simulink library "tp333079"  (Simulink 5.0)
values from neighbouring files (symbols this model uses):
  b = 1    [main_flock3.m]    (also in main_flock4.m; params_flocking_ros.m)
undefined symbols (not defined in the file or in its folder): AC, AlphaBnd, BetaBnd, CDda, CDde, CDdf, CDdr, CDM, CDmin, CGempty, CGgross, CL0, CLa, CLalphadot, Clbeta, Clda, CLde, CLdf, Cldr, CLM, CLmind, Clp, CLq, Clr, Cm0, Cma, Cmalphadot, Cmde, Cmdf, CmM, Cmq, Cnbeta, Cnda, Cndr, Cnp, Cnr, CP, CT, CYbeta, CYda, CYdr, CYp, CYr, Displacement, dmy, Engine, EulerIni, FuelFlow, FuelIni, J, Jempty, Jeng, Jgross, Jprop, MAC, MAP, MAPLim, MassIni, MaxPower, mempty ... (+26)
libraries: aerosimlib x325, simulink3 x42
(part 5 of 11)

== system tp333079/Transformations/Body-Inertial DCM From Euler Angles ==
  note: Sources
  note: Assemble Body-Inertial DCM
  note: Output
  note: Attitude trigonometry
  Euler : Inport  Port=1  PortDimensions=[3 1]  SampleTime=-1  DataType=auto
      settings: SignalType=auto
  -sin(theta) : Gain  Gain=-1  Multiplication=Element-wise(K.*u)  SaturateOnIntegerOverflow=on
  Demux : Demux  Outputs=3  BusSelectionMode=off
  Math Function : Math  Operator=transpose  OutputSignalType=auto
  Rbi Matrix : simulink3/Signals & Systems/Matrix Concatenation  numInports=3  catMethod=Horizontal
  Rbi Col1 : simulink3/Signals & Systems/Matrix Concatenation  numInports=3  catMethod=Vertical
  Rbi Col2 : simulink3/Signals & Systems/Matrix Concatenation  numInports=3  catMethod=Vertical
  Rbi Col3 : simulink3/Signals & Systems/Matrix Concatenation  numInports=3  catMethod=Vertical
  Sum2 : Sum  Inputs=+-  SaturateOnIntegerOverflow=on
  Sum3 : Sum  Inputs=++  SaturateOnIntegerOverflow=on
  Sum4 : Sum  Inputs=++  SaturateOnIntegerOverflow=on
  Sum5 : Sum  Inputs=+-  SaturateOnIntegerOverflow=on
  cos(phi) : Trigonometry  Operator=cos  OutputSignalType=auto
  cos(phi)cos(psi) : Product  Inputs=2  Multiplication=Element-wise(.*)  SaturateOnIntegerOverflow=on
  cos(phi)cos(theta) : Product  Inputs=2  Multiplication=Element-wise(.*)  SaturateOnIntegerOverflow=on
  cos(phi)sin(psi) : Product  Inputs=2  Multiplication=Element-wise(.*)  SaturateOnIntegerOverflow=on
  cos(phi)sin(theta)cos(psi) : Product  Inputs=3  Multiplication=Element-wise(.*)  SaturateOnIntegerOverflow=on
  cos(phi)sin(theta)sin(psi) : Product  Inputs=3  Multiplication=Element-wise(.*)  SaturateOnIntegerOverflow=on
  cos(psi) : Trigonometry  Operator=cos  OutputSignalType=auto
  cos(theta) : Trigonometry  Operator=cos  OutputSignalType=auto
  cos(theta)cos(psi) : Product  Inputs=2  Multiplication=Element-wise(.*)  SaturateOnIntegerOverflow=on
  cos(theta)sin(psi) : Product  Inputs=2  Multiplication=Element-wise(.*)  SaturateOnIntegerOverflow=on
  sin(phi) : Trigonometry  Operator=sin  OutputSignalType=auto
  sin(phi)cos(psi) : Product  Inputs=2  Multiplication=Element-wise(.*)  SaturateOnIntegerOverflow=on
  sin(phi)cos(theta) : Product  Inputs=2  Multiplication=Element-wise(.*)  SaturateOnIntegerOverflow=on
  sin(phi)sin(psi) : Product  Inputs=2  Multiplication=Element-wise(.*)  SaturateOnIntegerOverflow=on
  sin(phi)sin(theta)cos(psi) : Product  Inputs=3  Multiplication=Element-wise(.*)  SaturateOnIntegerOverflow=on
  sin(psi) : Trigonometry  Operator=sin  OutputSignalType=auto
  sin(theta) : Trigonometry  Operator=sin  OutputSignalType=auto
  DCM : Outport  Port=1
  wires:
  Euler/1 -> Demux/1
  Rbi Col1/1 -> Rbi Matrix/1
  Rbi Col2/1 -> Rbi Matrix/2
  Rbi Col3/1 -> Rbi Matrix/3
  Rbi Matrix/1 -> Math Function/1
  Demux/1 -> sin(phi)/1, cos(phi)/1
  Demux/2 -> cos(theta)/1, sin(theta)/1
  Demux/3 -> cos(psi)/1, sin(psi)/1
  sin(phi)/1 -> sin(phi)cos(psi)/1, sin(phi)sin(psi)/1, sin(phi)cos(theta)/1, sin(phi)sin(theta)cos(psi)/1
  cos(phi)/1 -> cos(phi)cos(theta)/1, cos(phi)sin(theta)sin(psi)/1, cos(phi)sin(theta)cos(psi)/1, cos(phi)cos(psi)/1, cos(phi)sin(psi)/1
  sin(theta)/1 -> cos(phi)sin(theta)cos(psi)/2, cos(phi)sin(theta)sin(psi)/2, sin(phi)sin(theta)cos(psi)/2, -sin(theta)/1
  cos(theta)/1 -> cos(phi)cos(theta)/2, sin(phi)cos(theta)/2, cos(theta)sin(psi)/1, cos(theta)cos(psi)/1
  sin(psi)/1 -> cos(phi)sin(theta)sin(psi)/3, sin(phi)sin(psi)/2, cos(phi)sin(psi)/2, cos(theta)sin(psi)/2
  cos(psi)/1 -> sin(phi)cos(psi)/2, cos(phi)sin(theta)cos(psi)/3, cos(phi)cos(psi)/2, sin(phi)sin(theta)cos(psi)/3, cos(theta)cos(psi)/2
  cos(phi)sin(psi)/1 -> Sum2/2
  cos(phi)cos(psi)/1 -> Sum3/2
  sin(phi)sin(theta)cos(psi)/1 -> Sum3/1, Sum2/1
  cos(phi)sin(theta)cos(psi)/1 -> Sum4/1
  sin(phi)sin(psi)/1 -> Sum4/2
  cos(phi)sin(theta)sin(psi)/1 -> Sum5/1
  sin(phi)cos(psi)/1 -> Sum5/2
  cos(theta)cos(psi)/1 -> Rbi Col1/1
  cos(theta)sin(psi)/1 -> Rbi Col1/2
  -sin(theta)/1 -> Rbi Col1/3
  Sum2/1 -> Rbi Col2/1
  Sum3/1 -> Rbi Col2/2
  sin(phi)cos(theta)/1 -> Rbi Col2/3
  Sum4/1 -> Rbi Col3/1
  Sum5/1 -> Rbi Col3/2
  cos(phi)cos(theta)/1 -> Rbi Col3/3
  Math Function/1 -> DCM/1

== system tp333079/Transformations/Body-Inertial DCM From Quaternions ==
  note: Output
  note: Quaternion products
  note: Assemble Body-Inertial DCM
  note: Sources
  Quaternions : Inport  Port=1  PortDimensions=[4 1]  SampleTime=-1  DataType=auto
      settings: SignalType=auto
  Demux : Demux  Outputs=4  BusSelectionMode=off
  Demux1 : Demux  Outputs=4  BusSelectionMode=off
  Gain{,1..5} (6 alike) : Gain  Gain=2  Multiplication=Element-wise(K.*u)  SaturateOnIntegerOverflow=on
  Get DCM : Math  Operator=transpose  OutputSignalType=auto
  Math Function : Math  Operator=square  OutputSignalType=auto
  Rbi Matrix : simulink3/Signals & Systems/Matrix Concatenation  numInports=3  catMethod=Horizontal
  Rbi Col1 : simulink3/Signals & Systems/Matrix Concatenation  numInports=3  catMethod=Vertical
  Rbi Col2 : simulink3/Signals & Systems/Matrix Concatenation  numInports=3  catMethod=Vertical
  Rbi Col3 : simulink3/Signals & Systems/Matrix Concatenation  numInports=3  catMethod=Vertical
  Sum : Sum  Inputs=++--  SaturateOnIntegerOverflow=on
  Sum1 : Sum  Inputs=++  SaturateOnIntegerOverflow=on
  Sum2 : Sum  Inputs=+-  SaturateOnIntegerOverflow=on
  Sum3 : Sum  Inputs=+-  SaturateOnIntegerOverflow=on
  Sum4 : Sum  Inputs=+-+-  SaturateOnIntegerOverflow=on
  Sum5 : Sum  Inputs=++  SaturateOnIntegerOverflow=on
  Sum6 : Sum  Inputs=++  SaturateOnIntegerOverflow=on
  Sum7 : Sum  Inputs=+-  SaturateOnIntegerOverflow=on
  Sum8 : Sum  Inputs=+--+  SaturateOnIntegerOverflow=on
  exe0 : Product  Inputs=2  Multiplication=Element-wise(.*)  SaturateOnIntegerOverflow=on
  exey : Product  Inputs=2  Multiplication=Element-wise(.*)  SaturateOnIntegerOverflow=on
  exez : Product  Inputs=2  Multiplication=Element-wise(.*)  SaturateOnIntegerOverflow=on
  eye0 : Product  Inputs=2  Multiplication=Element-wise(.*)  SaturateOnIntegerOverflow=on
  eyez : Product  Inputs=2  Multiplication=Element-wise(.*)  SaturateOnIntegerOverflow=on
  eze0 : Product  Inputs=2  Multiplication=Element-wise(.*)  SaturateOnIntegerOverflow=on
  DCM : Outport  Port=1
  wires:
  Get DCM/1 -> DCM/1
  Rbi Matrix/1 -> Get DCM/1
  Sum8/1 -> Rbi Col3/3
  Gain5/1 -> Rbi Col3/2
  Gain4/1 -> Rbi Col3/1
  Rbi Col3/1 -> Rbi Matrix/3
  Sum7/1 -> Gain5/1
  Sum6/1 -> Gain4/1
  Rbi Col2/1 -> Rbi Matrix/2
  Gain3/1 -> Rbi Col2/3
  Sum4/1 -> Rbi Col2/2
  Gain2/1 -> Rbi Col2/1
  Sum5/1 -> Gain3/1
  Sum3/1 -> Gain2/1
  Rbi Col1/1 -> Rbi Matrix/1
  Gain1/1 -> Rbi Col1/3
  Gain/1 -> Rbi Col1/2
  Sum/1 -> Rbi Col1/1
  Sum2/1 -> Gain1/1
  Sum1/1 -> Gain/1
  exe0/1 -> Sum5/2, Sum7/2
  eyez/1 -> Sum5/1, Sum7/1
  eye0/1 -> Sum2/2, Sum6/2
  exez/1 -> Sum2/1, Sum6/1
  eze0/1 -> Sum1/2, Sum3/2
  exey/1 -> Sum1/1, Sum3/1
  Math Function/1 -> Demux1/1
  Demux/4 -> eze0/1, exez/2, eyez/2
  Demux/3 -> exey/2, eye0/1, eyez/1
  Demux/2 -> exey/1, exez/1, exe0/1
  Demux/1 -> eze0/2, eye0/2, exe0/2
  Quaternions/1 -> Math Function/1, Demux/1
  Demux1/1 -> Sum/1, Sum4/1, Sum8/1
  Demux1/2 -> Sum/2, Sum4/2, Sum8/2
  Demux1/3 -> Sum/3, Sum4/3, Sum8/3
  Demux1/4 -> Sum/4, Sum4/4, Sum8/4

== system tp333079/Transformations/Body-Wind DCM ==
  note: Output
  note: Assemble Body-Wind DCM
  note: Trigonometric functions
  note: Sources
  WindAxesVel : Inport  Port=1  PortDimensions=[3 1]  SampleTime=-1  DataType=auto
      settings: SignalType=auto
  ChSign : Gain  Gain=-1  Multiplication=Element-wise(K.*u)  SaturateOnIntegerOverflow=on
  ChSign1 : Gain  Gain=-1  Multiplication=Element-wise(K.*u)  SaturateOnIntegerOverflow=on
  ChSign2 : Gain  Gain=-1  Multiplication=Element-wise(K.*u)  SaturateOnIntegerOverflow=on
  Demux : Demux  Outputs=3  BusSelectionMode=off
  Product{,1..3} (4 alike) : Product  Inputs=2  Multiplication=Element-wise(.*)  SaturateOnIntegerOverflow=on
  S Matrix : simulink3/Signals & Systems/Matrix Concatenation  numInports=3  catMethod=Horizontal
  S Col1 : simulink3/Signals & Systems/Matrix Concatenation  numInports=3  catMethod=Vertical
  S Col2 : simulink3/Signals & Systems/Matrix Concatenation  numInports=3  catMethod=Vertical
  S Col3 : simulink3/Signals & Systems/Matrix Concatenation  numInports=3  catMethod=Vertical
  Terminator : Terminator
  Trigonometric Function : Trigonometry  Operator=sin  OutputSignalType=auto
  Trigonometric Function1 : Trigonometry  Operator=cos  OutputSignalType=auto
  Trigonometric Function2 : Trigonometry  Operator=sin  OutputSignalType=auto
  Trigonometric Function3 : Trigonometry  Operator=cos  OutputSignalType=auto
  Zero : Constant  Value=0
  DCM : Outport  Port=1
  wires:
  S Matrix/1 -> DCM/1
  S Col3/1 -> S Matrix/3
  S Col2/1 -> S Matrix/2
  S Col1/1 -> S Matrix/1
  ChSign2/1 -> S Col3/2
  Product2/1 -> S Col3/1
  Product3/1 -> ChSign2/1
  Zero/1 -> S Col2/3
  ChSign1/1 -> S Col1/3
  ChSign/1 -> S Col1/2
  Product/1 -> S Col1/1
  Product1/1 -> ChSign/1
  Trigonometric Function3/1 -> Product/2, S Col2/2, Product2/2
  Trigonometric Function2/1 -> Product1/2, S Col2/1, Product3/2
  Trigonometric Function1/1 -> Product/1, Product1/1, S Col3/3
  Trigonometric Function/1 -> ChSign1/1, Product2/1, Product3/1
  Demux/1 -> Terminator/1
  WindAxesVel/1 -> Demux/1
  Demux/2 -> Trigonometric Function3/1, Trigonometric Function2/1
  Demux/3 -> Trigonometric Function/1, Trigonometric Function1/1

== system tp333079/Transformations/ECEF Position ==
  note: Trigonometric functions
  note: Sources
  note: Output
  LLA : Inport  Port=1  PortDimensions=[3 1]  SampleTime=-1  DataType=auto
      settings: SignalType=auto
  Demux : Demux  Outputs=3  BusSelectionMode=off
  Equatorial Radius : Constant  Value=6378137
  First Eccentricity : Constant  Value=0.0818191908426
  Mux : Mux  Inputs=3
  One : Constant  Value=1
  Product : Product  Inputs=3  Multiplication=Element-wise(.*)  SaturateOnIntegerOverflow=on
  Product1 : Product  Inputs=3  Multiplication=Element-wise(.*)  SaturateOnIntegerOverflow=on
  Product3 : Product  Inputs=2  Multiplication=Element-wise(.*)  SaturateOnIntegerOverflow=on
  Product4 : Product  Inputs=2  Multiplication=Element-wise(.*)  SaturateOnIntegerOverflow=on
  Product5 : Product  Inputs=*/  Multiplication=Element-wise(.*)  SaturateOnIntegerOverflow=on
  Product6 : Product  Inputs=2  Multiplication=Element-wise(.*)  SaturateOnIntegerOverflow=on
  Sum : Sum  Inputs=|++  SaturateOnIntegerOverflow=on
  Sum1 : Sum  Inputs=++|  SaturateOnIntegerOverflow=on
  Sum2 : Sum  Inputs=|+-  SaturateOnIntegerOverflow=on
  Sum3 : Sum  Inputs=|+-  SaturateOnIntegerOverflow=on
  Trigonometric Function : Trigonometry  Operator=sin  OutputSignalType=auto
  Trigonometric Function1 : Trigonometry  Operator=cos  OutputSignalType=auto
  Trigonometric Function2 : Trigonometry  Operator=sin  OutputSignalType=auto
  Trigonometric Function3 : Trigonometry  Operator=cos  OutputSignalType=auto
  eps^2 : Math  Operator=square  OutputSignalType=auto
  sin(phi)^2 : Math  Operator=square  OutputSignalType=auto
  sqrt : Math  Operator=sqrt  OutputSignalType=auto
  ECEF : Outport  Port=1
  wires:
  Mux/1 -> ECEF/1
  Product1/1 -> Mux/2
  Product/1 -> Mux/1
  Trigonometric Function3/1 -> Product/3
  Trigonometric Function2/1 -> Product1/3
  Trigonometric Function1/1 -> Product/2, Product1/2
  LLA/1 -> Demux/1
  Demux/1 -> Trigonometric Function1/1, Trigonometric Function/1
  Demux/2 -> Trigonometric Function2/1, Trigonometric Function3/1
  Product5/1 -> Product4/1, Sum1/2
  sqrt/1 -> Product5/2
  Equatorial Radius/1 -> Product5/1
  Sum3/1 -> sqrt/1
  Product6/1 -> Sum3/2
  sin(phi)^2/1 -> Product6/1
  Product4/1 -> Sum/2
  First Eccentricity/1 -> eps^2/1
  One/1 -> Sum3/1, Sum2/1
  eps^2/1 -> Product6/2, Sum2/2
  Sum2/1 -> Product4/2
  Sum/1 -> Product3/1
  Product3/1 -> Mux/3
  Demux/3 -> Sum1/1, Sum/1
  Sum1/1 -> Product/1, Product1/1
  Trigonometric Function/1 -> sin(phi)^2/1, Product3/2

== system tp333079/Transformations/Euler Angles From Quaternions ==
  note: Compute Euler angles
  note: Sources
  note: Quaternion products
  Quaternions : Inport  Port=1  PortDimensions=[4 1]  SampleTime=-1  DataType=auto
      settings: SignalType=auto
  2pi Bound : aerosimlib/Math/2pi Bound
  Demux : Demux  Outputs=4  BusSelectionMode=off
  Demux1 : Demux  Outputs=4  BusSelectionMode=off
  Gain6 : Gain  Gain=2  Multiplication=Element-wise(K.*u)  SaturateOnIntegerOverflow=on
  Gain7 : Gain  Gain=2  Multiplication=Element-wise(K.*u)  SaturateOnIntegerOverflow=on
  Gain8 : Gain  Gain=2  Multiplication=Element-wise(K.*u)  SaturateOnIntegerOverflow=on
  Math Function : Math  Operator=square  OutputSignalType=auto
  Mux : Mux  Inputs=3
  Sum10 : Sum  Inputs=+--+  SaturateOnIntegerOverflow=on
  Sum11 : Sum  Inputs=-+  SaturateOnIntegerOverflow=on
  Sum12 : Sum  Inputs=++  SaturateOnIntegerOverflow=on
  Sum13 : Sum  Inputs=++--  SaturateOnIntegerOverflow=on
  Sum9 : Sum  Inputs=++  SaturateOnIntegerOverflow=on
  Trigonometric Function : Trigonometry  Operator=atan2  OutputSignalType=auto
  Trigonometric Function1 : Trigonometry  Operator=asin  OutputSignalType=auto
  Trigonometric Function2 : Trigonometry  Operator=atan2  OutputSignalType=auto
  exe0 : Product  Inputs=2  Multiplication=Element-wise(.*)  SaturateOnIntegerOverflow=on
  exey : Product  Inputs=2  Multiplication=Element-wise(.*)  SaturateOnIntegerOverflow=on
  exez : Product  Inputs=2  Multiplication=Element-wise(.*)  SaturateOnIntegerOverflow=on
  eye0 : Product  Inputs=2  Multiplication=Element-wise(.*)  SaturateOnIntegerOverflow=on
  eyez : Product  Inputs=2  Multiplication=Element-wise(.*)  SaturateOnIntegerOverflow=on
  eze0 : Product  Inputs=2  Multiplication=Element-wise(.*)  SaturateOnIntegerOverflow=on
  pi Bound : aerosimlib/Math/pi Bound
  pi Bound1 : aerosimlib/Math/pi Bound
  Euler : Outport  Port=1
  wires:
  Sum9/1 -> Gain6/1
  Gain6/1 -> Trigonometric Function/1
  Sum10/1 -> Trigonometric Function/2
  Sum11/1 -> Gain7/1
  Gain7/1 -> Trigonometric Function1/1
  Sum12/1 -> Gain8/1
  Gain8/1 -> Trigonometric Function2/1
  Sum13/1 -> Trigonometric Function2/2
  Trigonometric Function1/1 -> pi Bound1/1
  Trigonometric Function/1 -> pi Bound/1
  Trigonometric Function2/1 -> 2pi Bound/1
  Quaternions/1 -> Math Function/1, Demux/1
  Demux/1 -> eze0/2, eye0/2, exe0/2
  Demux/2 -> exey/1, exez/1, exe0/1
  Demux/3 -> exey/2, eye0/1, eyez/1
  Demux/4 -> eze0/1, exez/2, eyez/2
  Demux1/1 -> Sum10/1, Sum13/1
  Demux1/2 -> Sum10/2, Sum13/2
  Demux1/3 -> Sum10/3, Sum13/3
  Demux1/4 -> Sum10/4, Sum13/4
  Math Function/1 -> Demux1/1
  exey/1 -> Sum12/1
  eze0/1 -> Sum12/2
  exez/1 -> Sum11/1
  eye0/1 -> Sum11/2
  eyez/1 -> Sum9/1
  exe0/1 -> Sum9/2
  Mux/1 -> Euler/1
  pi Bound/1 -> Mux/1
  pi Bound1/1 -> Mux/2
  2pi Bound/1 -> Mux/3

== system tp333079/Transformations/Euler Angles  From DCM ==
  DCM : Inport  Port=1  PortDimensions=[3 3]  SampleTime=-1  DataType=auto
      settings: SignalType=auto
  C12 : Selector  InputType=Matrix  ElementSrc=Internal  Elements=[1 3]  RowSrc=Internal  Rows=1  ColumnSrc=Internal  Columns=2  InputPortWidth=3
  C13 : Selector  InputType=Matrix  ElementSrc=Internal  Elements=[1 3]  RowSrc=Internal  Rows=1  ColumnSrc=Internal  Columns=3  InputPortWidth=3
  C23 : Selector  InputType=Matrix  ElementSrc=Internal  Elements=[1 3]  RowSrc=Internal  Rows=2  ColumnSrc=Internal  Columns=3  InputPortWidth=3
  ChSign : Gain  Gain=-1  Multiplication=Element-wise(K.*u)  SaturateOnIntegerOverflow=on
  Mux3 : Mux  Inputs=3
  Product2 : Product  Inputs=*/  Multiplication=Element-wise(.*)  SaturateOnIntegerOverflow=on
  Product3 : Product  Inputs=*/  Multiplication=Element-wise(.*)  SaturateOnIntegerOverflow=on
  Trigonometric Function : Trigonometry  Operator=asin  OutputSignalType=auto
  Trigonometric Function1 : Trigonometry  Operator=cos  OutputSignalType=auto
  Trigonometric Function2 : Trigonometry  Operator=asin  OutputSignalType=auto
  Trigonometric Function3 : Trigonometry  Operator=asin  OutputSignalType=auto
  Euler : Outport  Port=1
  wires:
  DCM/1 -> C12/1, C23/1, C13/1
  Mux3/1 -> Euler/1
  Trigonometric Function3/1 -> Mux3/1
  Trigonometric Function2/1 -> Mux3/3
  Product2/1 -> Trigonometric Function2/1
  Product3/1 -> Trigonometric Function3/1
  C23/1 -> Product3/1
  Trigonometric Function1/1 -> Product3/2, Product2/2
  C12/1 -> Product2/1
  Trigonometric Function/1 -> Mux3/2, Trigonometric Function1/1
  ChSign/1 -> Trigonometric Function/1
  C13/1 -> ChSign/1

== system tp333079/Transformations/Quaternions From Euler Angles ==
  note: Sources
  note: Attitude trigonometry
  note: Compute quaternions
  note: Outputs
  Euler : Inport  Port=1  PortDimensions=[3 1]  SampleTime=-1  DataType=auto
      settings: SignalType=auto
  1/2 : Gain  Gain=1/2  Multiplication=Element-wise(K.*u)  SaturateOnIntegerOverflow=on
  CCC : Product  Inputs=3  Multiplication=Element-wise(.*)  SaturateOnIntegerOverflow=on
  CCS : Product  Inputs=3  Multiplication=Element-wise(.*)  SaturateOnIntegerOverflow=on
  CSC : Product  Inputs=3  Multiplication=Element-wise(.*)  SaturateOnIntegerOverflow=on
  CSS : Product  Inputs=3  Multiplication=Element-wise(.*)  SaturateOnIntegerOverflow=on
  Demux : Demux  Outputs=3  BusSelectionMode=off
  Mux : Mux  Inputs=4
  SCC : Product  Inputs=3  Multiplication=Element-wise(.*)  SaturateOnIntegerOverflow=on
  SCS : Product  Inputs=3  Multiplication=Element-wise(.*)  SaturateOnIntegerOverflow=on
  SSC : Product  Inputs=3  Multiplication=Element-wise(.*)  SaturateOnIntegerOverflow=on
  SSS : Product  Inputs=3  Multiplication=Element-wise(.*)  SaturateOnIntegerOverflow=on
  Sum1 : Sum  Inputs=++  SaturateOnIntegerOverflow=on
  Sum2 : Sum  Inputs=+-  SaturateOnIntegerOverflow=on
  Sum3 : Sum  Inputs=+-  SaturateOnIntegerOverflow=on
  Sum9 : Sum  Inputs=++  SaturateOnIntegerOverflow=on
  cos(phi/2) : Trigonometry  Operator=cos  OutputSignalType=auto
  cos(psi/2) : Trigonometry  Operator=cos  OutputSignalType=auto
  cos(theta/2) : Trigonometry  Operator=cos  OutputSignalType=auto
  sin(phi/2) : Trigonometry  Operator=sin  OutputSignalType=auto
  sin(psi/2) : Trigonometry  Operator=sin  OutputSignalType=auto
  sin(theta/2) : Trigonometry  Operator=sin  OutputSignalType=auto
  Quaternions : Outport  Port=1
  wires:
  Mux/1 -> Quaternions/1
  Euler/1 -> 1/2/1
  1/2/1 -> Demux/1
  Demux/1 -> sin(phi/2)/1, cos(phi/2)/1
  Demux/2 -> cos(theta/2)/1, sin(theta/2)/1
  Demux/3 -> cos(psi/2)/1, sin(psi/2)/1
  cos(psi/2)/1 -> CCC/3, SCC/3, SSC/3, CSC/3
  sin(psi/2)/1 -> SSS/3, CSS/3, CCS/3, SCS/3
  cos(theta/2)/1 -> SCC/2, CCS/2, SCS/2, CCC/2
  sin(theta/2)/1 -> SSS/2, CSS/2, SSC/2, CSC/2
  cos(phi/2)/1 -> CSS/1, CCS/1, CSC/1, CCC/1
  sin(phi/2)/1 -> SCC/1, SSC/1, SCS/1, SSS/1
  CCC/1 -> Sum9/1
  SSS/1 -> Sum9/2
  CSC/1 -> Sum1/1
  SCS/1 -> Sum1/2
  SCC/1 -> Sum2/1
  CSS/1 -> Sum2/2
  CCS/1 -> Sum3/1
  SSC/1 -> Sum3/2
  Sum9/1 -> Mux/1
  Sum2/1 -> Mux/2
  Sum1/1 -> Mux/3
  Sum3/1 -> Mux/4

== system tp333079/Unit Conversion/Angular position ==
  deg 2 rad : Subsystem  SimViewingDevice=off
      settings: Permissions=ReadWrite  RTWFcnNameOpts=Auto  RTWFileNameOpts=Auto
      mask Type: Deg to rad
      mask Description: Convert degrees to radians.
      mask Help:
      | Degrees to radians conversion.
      | <P><B>Input:</B> angle in degrees;</P>
      | <P><B>Output:</B> angle in radians.</P>
      mask Display: disp('DEG RAD');
  rad 2 deg : Subsystem  SimViewingDevice=off
      settings: Permissions=ReadWrite  RTWFcnNameOpts=Auto  RTWFileNameOpts=Auto
      mask Type: Radians to degrees
      mask Description: Convert radians to degrees.
      mask Help:
      | Radians to degrees conversion.
      | <P><B>Input:</B> angle in radians;</P>
      | <P><B>Output:</B> angle in degrees.</P>
      mask Display: disp('RAD DEG');

== system tp333079/Unit Conversion/Angular velocity ==
  RPM 2 rad/s : Subsystem  SimViewingDevice=off
      settings: Permissions=ReadWrite  RTWFcnNameOpts=Auto  RTWFileNameOpts=Auto
      mask Type: RPM to rad/s
      mask Description: Convert rotations-per-minute to radians-per-second.
      mask Help:
      | Rotations per minute to radians per second conversion.
      | <P><B>Input:</B> angular speed in rotations per minute;</P>
      | <P><B>Output:</B> angular speed in radians per second.</P>
  rad/s 2 RPM : Subsystem  SimViewingDevice=off
      settings: Permissions=ReadWrite  RTWFcnNameOpts=Auto  RTWFileNameOpts=Auto
      mask Type: rad/s to RPM
      mask Description: Convert radians-per-second to rotations-per-minute.
      mask Help:
      | Radians per second to rotations per minute conversion.
      | <P><B>Input:</B> angular speed in radians per second;</P>
      | <P><B>Output:</B> angular speed in rotations per minute.</P>

== system tp333079/Unit Conversion/Distance ==
  ft 2 m : Subsystem  SimViewingDevice=off
      settings: Permissions=ReadWrite  RTWFcnNameOpts=Auto  RTWFileNameOpts=Auto
      mask Type: Feet to meters
      mask Description: Convert feet to meters.
      mask Help:
      | Feet to meters conversion.
      | <P><B>Input:</B> distance in feet;</P>
      | <P><B>Output:</B> distance in meters.</P>
      mask Display: disp('FT       M');
  m 2 ft : Subsystem  SimViewingDevice=off
      settings: Permissions=ReadWrite  RTWFcnNameOpts=Auto  RTWFileNameOpts=Auto
      mask Type: Meters to feet
      mask Description: Convert meters to feet.
      mask Help:
      | Meters to feet conversion.
      | <P><B>Input:</B> distance in meters;</P>
      | <P><B>Output:</B> distance in feet.</P>
      mask Display: disp('M       FT');
  m 2 nm : Subsystem  SimViewingDevice=off
      settings: Permissions=ReadWrite  RTWFcnNameOpts=Auto  RTWFileNameOpts=Auto
      mask Type: Meters to nautical miles
      mask Description: Convert meters to nautical miles.
      mask Help:
      | Meters to nautical miles conversion.
      | <P><B>Input:</B> distance in meters;</P>
      | <P><B>Output:</B> distance in nautical miles.</P>
      mask Display: disp('M       NM');
  nm 2 m : Subsystem  SimViewingDevice=off
      settings: Permissions=ReadWrite  RTWFcnNameOpts=Auto  RTWFileNameOpts=Auto
      mask Type: Nautical miles to meters
      mask Description: Convert nautical miles to meters.
      mask Help:
      | Nautical miles to meters conversion.
      | <P><B>Input:</B> distance in nautical miles;</P>
      | <P><B>Output:</B> distance in meters.</P>
      mask Display: disp('NM       M');

== system tp333079/Unit Conversion/Force ==
  N 2 lbf : Subsystem  SimViewingDevice=off
      settings: Permissions=ReadWrite  RTWFcnNameOpts=Auto  RTWFileNameOpts=Auto
      mask Type: Newtons to pounds
      mask Description: Convert newtons to pounds-force.
      mask Help:
      | Newton to pound conversion.
      | <P><B>Input:</B> force in newtons;</P>
      | <P><B>Output:</B> force in pounds.</P>
      mask Display: disp('N       lbf');
  lbf 2 N : Subsystem  SimViewingDevice=off
      settings: Permissions=ReadWrite  RTWFcnNameOpts=Auto  RTWFileNameOpts=Auto
      mask Type: Pounds to newtons
      mask Description: Convert pounds-force to newtons.
      mask Help:
      | Pound to newton conversion.
      | <P><B>Input:</B> force in pounds;</P>
      | <P><B>Output:</B> force in newtons.</P>
      mask Display: disp('lbf       N');

== system tp333079/Unit Conversion/Mass ==
  kg 2 lb : Subsystem  SimViewingDevice=off
      settings: Permissions=ReadWrite  RTWFcnNameOpts=Auto  RTWFileNameOpts=Auto
      mask Type: Kilograms to pounds
      mask Description: Convert kilograms to pounds.
      mask Help:
      | Kilograms to pounds conversion.
      | <P><B>Input:</B> mass in kilograms;</P>
      | <P><B>Output:</B> weight in pounds (at sea-level).</P>
      mask Display: disp(['__________';'          ';'KG        ';'        LB';'g         ';'----------']);
  kg 2 slug : Subsystem  SimViewingDevice=off
      settings: Permissions=ReadWrite  RTWFcnNameOpts=Auto  RTWFileNameOpts=Auto
      mask Type: Kilograms to slugs
      mask Description: Convert kilograms to slugs.
      mask Help:
      | Kilogram to slug conversion.
      | <P><B>Input:</B> mass in kilograms;</P>
      | <P><B>Output:</B> mass in slugs.</P>
      mask Display: disp('kg     slug');
  lb 2 kg : Subsystem  SimViewingDevice=off
      settings: Permissions=ReadWrite  RTWFcnNameOpts=Auto  RTWFileNameOpts=Auto
      mask Type: Pounds to kilograms
      mask Description: Convert pounds to kilograms.
      mask Help:
      | Pounds to kilograms conversion.
      | <P><B>Input:</B> weight in pounds (at sea-level);</P>
      | <P><B>Output:</B> mass in kilograms.</P>
      mask Display: disp(['__________';'          ';'LB        ';'        KG';'g         ';'----------']);
  slug 2 kg : Subsystem  SimViewingDevice=off
      settings: Permissions=ReadWrite  RTWFcnNameOpts=Auto  RTWFileNameOpts=Auto
      mask Type: Slugs to kilograms
      mask Description: Convert slugs to kilograms.
      mask Help:
      | Slug to kilogram conversion.
      | <P><B>Input:</B> mass in slugs;</P>
      | <P><B>Output:</B> mass in kilograms.</P>
      mask Display: disp('slug     kg');

== system tp333079/Unit Conversion/Pressure ==
  Pa2inHg : Subsystem  SimViewingDevice=off
      settings: Permissions=ReadWrite  RTWFcnNameOpts=Auto  RTWFileNameOpts=Auto
      mask Type: Pa to in.Hg
      mask Description: Convert pressure from Pascals to inches Hg.
      mask Help:
      | Convert pressure from Pascals to inches Hg.
      | <P><B>Input:</B> pressure in Pascals;</P>
      | <P><B>Output:</B> pressure in inches Hg.</P>
  inHg2Pa : Subsystem  SimViewingDevice=off
      settings: Permissions=ReadWrite  RTWFcnNameOpts=Auto  RTWFileNameOpts=Auto
      mask Type: in. Hg to Pa
      mask Description: Convert pressure from inches Hg to Pascals.
      mask Help:
      | Convert pressure from inches Hg to Pascals.
      | <P><B>Input:</B> pressure in inches Hg;</P>
      | <P><B>Output:</B> pressure in Pascals.</P>

== system tp333079/Unit Conversion/Temperature ==
  F2K : Subsystem  SimViewingDevice=off
      settings: Permissions=ReadWrite  RTWFcnNameOpts=Auto  RTWFileNameOpts=Auto
      mask Type: Degrees F to degrees K
      mask Description: Convert temperature from degrees Fahrenheit to degrees Kelvin.
      mask Help:
      | Convert temperature from degrees Fahrenheit to degrees Kelvin.
      | <P><B>Input:</B> temperature in degrees Fahrenheit;</P>
      | <P><B>Output:</B> temperature in degrees Kelvin.</P>
  K2F : Subsystem  SimViewingDevice=off
      settings: Permissions=ReadWrite  RTWFcnNameOpts=Auto  RTWFileNameOpts=Auto
      mask Type: Degrees K to degrees F
      mask Description: Convert temperature from degrees Kelvin to degrees Fahrenheit.
      mask Help:
      | Convert temperature from degrees Kelvin to degrees Fahrenheit.
      | <P><B>Input:</B> temperature in degrees Kelvin;</P>
      | <P><B>Output:</B> temperature in degrees Fahrenheit.</P>

== system tp333079/Unit Conversion/Velocity ==
  km/h 2 m/s : Subsystem  SimViewingDevice=off
      settings: Permissions=ReadWrite  RTWFcnNameOpts=Auto  RTWFileNameOpts=Auto
      mask Type: Kilometers per hour to meters per second
      mask Description: Convert kilometers per hour to meters per second.
      mask Help:
      | Kilometers per hour to meters per second conversion.
      | <P><B>Input:</B> speed in kilometers per hour;</P>
      | <P><B>Output:</B> speed in meters per second.</P>
      mask Display: disp('KM/H M/S');
  kts 2 m/s : Subsystem  SimViewingDevice=off
      settings: Permissions=ReadWrite  RTWFcnNameOpts=Auto  RTWFileNameOpts=Auto
      mask Type: Knots to meters per second
      mask Description: Convert knots to meters per second.
      mask Help:
      | Knots to meters per second conversion.
      | <P><B>Input:</B> speed in knots;</P>
      | <P><B>Output:</B> speed in meters per second.</P>
      mask Display: disp('KTS  M/S');
  m/s 2 km/h : Subsystem  SimViewingDevice=off
      settings: Permissions=ReadWrite  RTWFcnNameOpts=Auto  RTWFileNameOpts=Auto
      mask Type: Meters per second to kilometers per hour
      mask Description: Convert meters per second to kilometers per hour.
      mask Help:
      | Meters per second to kilometers per hour conversion.
      | <P><B>Input:</B> speed in meters per second;</P>
      | <P><B>Output:</B> speed in kilometers per hour.</P>
      mask Display: disp('M/S KM/H');
  m/s 2 kts : Subsystem  SimViewingDevice=off
      settings: Permissions=ReadWrite  RTWFcnNameOpts=Auto  RTWFileNameOpts=Auto
      mask Type: Meters per second to knots
      mask Description: Convert meters per second to knots.
      mask Help:
      | Meters per second to knots conversion.
      | <P><B>Input:</B> speed in meters per second;</P>
      | <P><B>Output:</B> speed in knots.</P>
      mask Display: disp('M/S  KTS');
  m/s 2 mph : Subsystem  SimViewingDevice=off
      settings: Permissions=ReadWrite  RTWFcnNameOpts=Auto  RTWFileNameOpts=Auto
      mask Type: Meters per second to miles per hour
      mask Description: Convert meters per second to miles per hour.
      mask Help:
      | Meters per second to miles per hour conversion.
      | <P><B>Input:</B> speed in meters per second;</P>
      | <P><B>Output:</B> speed in miles per hour.</P>
      mask Display: disp('M/S MPH');
  mph 2 m/s : Subsystem  SimViewingDevice=off
      settings: Permissions=ReadWrite  RTWFcnNameOpts=Auto  RTWFileNameOpts=Auto
      mask Type: Miles per hour to meters per second
      mask Description: Convert miles per hour to meters per second.
      mask Help:
      | Miles per hour to meters per second conversion.
      | <P><B>Input:</B> speed in miles per hour;</P>
      | <P><B>Output:</B> speed in meters per second.</P>
      mask Display: disp('MPH M/S');

== system tp333079/Unit Conversion/Volume ==
  gal 2 l : Subsystem  SimViewingDevice=off
      settings: Permissions=ReadWrite  RTWFcnNameOpts=Auto  RTWFileNameOpts=Auto
      mask Type: Gallons to liters
      mask Description: Convert gallons to liters.
      mask Help:
      | Gallon to liter conversion.
      | <P><B>Input:</B> volume in gallons;</P>
      | <P><B>Output:</B> volume in liters.</P>
      mask Display: disp('gal       l');
  l 2 gal : Subsystem  SimViewingDevice=off
      settings: Permissions=ReadWrite  RTWFcnNameOpts=Auto  RTWFileNameOpts=Auto
      mask Type: Liters to gallons
      mask Description: Convert liters to gallons.
      mask Help:
      | Liter to gallon conversion.
      | <P><B>Input:</B> volume in liters;</P>
      | <P><B>Output:</B> volume in gallons.</P>
      mask Display: disp('l       gal');

== system tp333079/Atmosphere/Turbulence/Lateral  Turbulence Filter ==
  note: Outputs
  note: Filter dynamics
  note: Build state space model
  note: Matrix elements
  note: Sources
  Airspeed : Inport  Port=1  PortDimensions=1  SampleTime=-1  DataType=auto
      settings: SignalType=auto
  RefLength : Inport  Port=2  PortDimensions=1  SampleTime=-1  DataType=auto
      settings: SignalType=auto
  Intensity : Inport  Port=3  PortDimensions=1  SampleTime=-1  DataType=auto
      settings: SignalType=auto
  A : simulink3/Signals & Systems/Matrix Concatenation  numInports=2  catMethod=Vertical
  A row 1 : simulink3/Signals & Systems/Matrix Concatenation  numInports=2  catMethod=Horizontal
  A row 2 : simulink3/Signals & Systems/Matrix Concatenation  numInports=2  catMethod=Horizontal
  Ax : Product  Inputs=2  Multiplication=Matrix(*)  SaturateOnIntegerOverflow=on
  B : simulink3/Signals & Systems/Matrix Concatenation  numInports=2  catMethod=Vertical
  Bu : Product  Inputs=2  Multiplication=Matrix(*)  SaturateOnIntegerOverflow=on
  C : simulink3/Signals & Systems/Matrix Concatenation  numInports=2  catMethod=Horizontal
  Constant : Constant  Value=0
  Constant1 : Constant  Value=1
  Cx : Product  Inputs=2  Multiplication=Matrix(*)  SaturateOnIntegerOverflow=on
  Derivative : Derivative
  Gain : Gain  Gain=2  Multiplication=Element-wise(K.*u)  SaturateOnIntegerOverflow=on
  Gain1 : Gain  Gain=-28.84  Multiplication=Element-wise(K.*u)  SaturateOnIntegerOverflow=on
  Gain2 : Gain  Gain=1.776  Multiplication=Element-wise(K.*u)  SaturateOnIntegerOverflow=on
  Gain3 : Gain  Gain=-26.51  Multiplication=Element-wise(K.*u)  SaturateOnIntegerOverflow=on
  Gain4 : Gain  Gain=26.51  Multiplication=Element-wise(K.*u)  SaturateOnIntegerOverflow=on
  Integrator : Integrator  ExternalReset=none  InitialConditionSource=internal  InitialCondition=zeros(2,1)  LimitOutput=off  UpperSaturationLimit=inf  LowerSaturationLimit=-inf  ShowSaturationPort=off  ShowStatePort=off  AbsoluteTolerance=auto
  Math Function : Math  Operator=square  OutputSignalType=auto
  Math Function1 : Math  Operator=sqrt  OutputSignalType=auto
  Product : Product  Inputs=*/  Multiplication=Element-wise(.*)  SaturateOnIntegerOverflow=on
  Product1 : Product  Inputs=*/  Multiplication=Element-wise(.*)  SaturateOnIntegerOverflow=on
  Product2 : Product  Inputs=2  Multiplication=Element-wise(.*)  SaturateOnIntegerOverflow=on
  Sum : Sum  Inputs=|++  SaturateOnIntegerOverflow=on
  White Noise : RandomNumber  Mean=0  Variance=1  Seed=[32412]  SampleTime=tsamp
  LatVel : Outport  Port=1
  LatAcc : Outport  Port=2
  wires:
  Integrator/1 -> Cx/2, Ax/2
  Intensity/1 -> Product2/2
  Derivative/1 -> LatAcc/1
  Cx/1 -> Derivative/1, LatVel/1
  Bu/1 -> Sum/2
  White Noise/1 -> Bu/2
  Sum/1 -> Integrator/1
  Ax/1 -> Sum/1
  C/1 -> Cx/1
  B/1 -> Bu/1
  A/1 -> Ax/1
  A row 2/1 -> A/2
  A row 1/1 -> A/1
  Constant/1 -> B/2, A row 2/2
  Constant1/1 -> A row 2/1
  Product2/1 -> B/1
  Math Function1/1 -> Product2/1
  Gain4/1 -> C/2
  Gain3/1 -> A row 1/2
  Math Function/1 -> Gain4/1, Gain3/1
  Gain2/1 -> C/1
  Gain1/1 -> A row 1/1
  Gain/1 -> Math Function1/1
  Product/1 -> Gain2/1, Gain1/1, Math Function/1
  Product1/1 -> Gain/1
  RefLength/1 -> Product/2, Product1/1
  Airspeed/1 -> Product/1, Product1/2

== system tp333079/Atmosphere/Turbulence/Longitudinal  Turbulence Filter ==
  note: Sources
  note: Matrix elements
  note: Build state space model
  note: Filter dynamics
  note: Outputs
  Airspeed : Inport  Port=1  PortDimensions=1  SampleTime=-1  DataType=auto
      settings: SignalType=auto
  RefLength : Inport  Port=2  PortDimensions=1  SampleTime=-1  DataType=auto
      settings: SignalType=auto
  Intensity : Inport  Port=3  PortDimensions=1  SampleTime=-1  DataType=auto
      settings: SignalType=auto
  A : simulink3/Signals & Systems/Matrix Concatenation  numInports=2  catMethod=Vertical
  A row 1 : simulink3/Signals & Systems/Matrix Concatenation  numInports=2  catMethod=Horizontal
  A row 2 : simulink3/Signals & Systems/Matrix Concatenation  numInports=2  catMethod=Horizontal
  Ax : Product  Inputs=2  Multiplication=Matrix(*)  SaturateOnIntegerOverflow=on
  B : simulink3/Signals & Systems/Matrix Concatenation  numInports=2  catMethod=Vertical
  Bu : Product  Inputs=2  Multiplication=Matrix(*)  SaturateOnIntegerOverflow=on
  C : simulink3/Signals & Systems/Matrix Concatenation  numInports=2  catMethod=Horizontal
  Constant : Constant  Value=0
  Constant1 : Constant  Value=1
  Cx : Product  Inputs=2  Multiplication=Matrix(*)  SaturateOnIntegerOverflow=on
  Derivative : Derivative
  Gain : Gain  Gain=2  Multiplication=Element-wise(K.*u)  SaturateOnIntegerOverflow=on
  Gain1 : Gain  Gain=-28.84  Multiplication=Element-wise(K.*u)  SaturateOnIntegerOverflow=on
  Gain2 : Gain  Gain=1.776  Multiplication=Element-wise(K.*u)  SaturateOnIntegerOverflow=on
  Gain3 : Gain  Gain=-26.51  Multiplication=Element-wise(K.*u)  SaturateOnIntegerOverflow=on
  Gain4 : Gain  Gain=26.51  Multiplication=Element-wise(K.*u)  SaturateOnIntegerOverflow=on
  Integrator : Integrator  ExternalReset=none  InitialConditionSource=internal  InitialCondition=zeros(2,1)  LimitOutput=off  UpperSaturationLimit=inf  LowerSaturationLimit=-inf  ShowSaturationPort=off  ShowStatePort=off  AbsoluteTolerance=auto
  Math Function : Math  Operator=square  OutputSignalType=auto
  Math Function1 : Math  Operator=sqrt  OutputSignalType=auto
  Product : Product  Inputs=*/  Multiplication=Element-wise(.*)  SaturateOnIntegerOverflow=on
  Product1 : Product  Inputs=*/  Multiplication=Element-wise(.*)  SaturateOnIntegerOverflow=on
  Product2 : Product  Inputs=2  Multiplication=Element-wise(.*)  SaturateOnIntegerOverflow=on
  Sum : Sum  Inputs=|++  SaturateOnIntegerOverflow=on
  White Noise : RandomNumber  Mean=0  Variance=1  Seed=[12344]  SampleTime=tsamp
  LongVel : Outport  Port=1
  LongAcc : Outport  Port=2
  wires:
  Airspeed/1 -> Product1/2, Product/1
  RefLength/1 -> Product1/1, Product/2
  Product1/1 -> Gain/1
  Product/1 -> Math Function/1, Gain1/1, Gain2/1
  Gain/1 -> Math Function1/1
  Gain1/1 -> A row 1/1
  Gain2/1 -> C/1
  Math Function/1 -> Gain3/1, Gain4/1
  Gain3/1 -> A row 1/2
  Gain4/1 -> C/2
  Math Function1/1 -> Product2/1
  Product2/1 -> B/1
  Constant1/1 -> A row 2/1
  Constant/1 -> A row 2/2, B/2
  A row 1/1 -> A/1
  A row 2/1 -> A/2
  A/1 -> Ax/1
  B/1 -> Bu/1
  C/1 -> Cx/1
  Ax/1 -> Sum/1
  Sum/1 -> Integrator/1
  White Noise/1 -> Bu/2
  Bu/1 -> Sum/2
  Cx/1 -> LongVel/1, Derivative/1
  Derivative/1 -> LongAcc/1
  Intensity/1 -> Product2/2
  Integrator/1 -> Ax/2, Cx/2

== system tp333079/Atmosphere/Turbulence/Turbulence Characteristics ==
  note: Sources
  note: Outputs
  AGLAlt : Inport  Port=1  PortDimensions=1  SampleTime=-1  DataType=auto
      settings: SignalType=auto
  WindVel : Inport  Port=2  PortDimensions=[3 1]  SampleTime=-1  DataType=auto
      settings: SignalType=auto
  Constant : Constant  Value=0.177
  Constant1 : Constant  Value=0.4
  Constant2 : Constant  Value=1.2
  Constant3 : Constant  Value=75.6
  Constant4 : Constant  Value=10
  Constant5 : Constant  Value=1000
  Gain : Gain  Gain=0.1  Multiplication=Element-wise(K.*u)  SaturateOnIntegerOverflow=on
  Gain1 : Gain  Gain=0.000823  Multiplication=Element-wise(K.*u)  SaturateOnIntegerOverflow=on
  Math Function : Math  Operator=pow  OutputSignalType=auto
  Math Function1 : Math  Operator=pow  OutputSignalType=auto
  Product : Product  Inputs=*/  Multiplication=Element-wise(.*)  SaturateOnIntegerOverflow=on
  Product1 : Product  Inputs=*/  Multiplication=Element-wise(.*)  SaturateOnIntegerOverflow=on
  Sum : Sum  Inputs=|++  SaturateOnIntegerOverflow=on
  Switch : Switch  Threshold=1000
  Switch1 : Switch  Threshold=1000
  Switch2 : Switch  Threshold=1000
  Switch3 : Switch  Threshold=10
  Switch4 : Switch  Threshold=10
  Switch5 : Switch  Threshold=10
  Vector norm : Subsystem  SimViewingDevice=off
      settings: Permissions=ReadWrite  RTWFcnNameOpts=Auto  RTWFileNameOpts=Auto
      mask Type: Vector norm-2
      mask Description: Compute the 2-norm (magnitude) of a vector, |v| = sqrt(v'v).
  sigmau : Outport  Port=1
  sigmav : Outport  Port=2
  sigmaw : Outport  Port=3
  Lu : Outport  Port=4
  Lv : Outport  Port=5
  Lw : Outport  Port=6
  wires:
  AGLAlt/1 -> Switch/2, Switch1/2, Switch2/2, Switch3/2, Switch4/2, Switch5/2, Switch5/1, Product1/1, Gain1/1
  WindVel/1 -> Vector norm/1(Vec)
  Gain/1 -> Product/1, sigmaw/1
  Constant/1 -> Sum/1
  Gain1/1 -> Sum/2
  Sum/1 -> Math Function/1, Math Function1/1
  Constant1/1 -> Math Function/2
  Constant2/1 -> Math Function1/2
  Constant4/1 -> Switch5/3
  Constant5/1 -> Switch2/1, Switch1/1, Switch/1
  Switch3/1 -> Switch/3
  Switch4/1 -> Switch1/3
  Switch5/1 -> Switch2/3
  Switch/1 -> Lu/1
  Switch1/1 -> Lv/1
  Switch2/1 -> Lw/1
  Product1/1 -> Switch3/1, Switch4/1
  Constant3/1 -> Switch4/3, Switch3/3
  Math Function/1 -> Product/2
  Math Function1/1 -> Product1/2
  Vector norm/1(Mag) -> Gain/1
  Product/1 -> sigmau/1, sigmav/1

== system tp333079/Atmosphere/Turbulence/Vertical  Turbulence Filter ==
  note: Sources
  note: Matrix elements
  note: Build state space model
  note: Filter dynamics
  note: Outputs
  Airspeed : Inport  Port=1  PortDimensions=1  SampleTime=-1  DataType=auto
      settings: SignalType=auto
  RefLength : Inport  Port=2  PortDimensions=1  SampleTime=-1  DataType=auto
      settings: SignalType=auto
  Intensity : Inport  Port=3  PortDimensions=1  SampleTime=-1  DataType=auto
      settings: SignalType=auto
  A : simulink3/Signals & Systems/Matrix Concatenation  numInports=2  catMethod=Vertical
  A row 1 : simulink3/Signals & Systems/Matrix Concatenation  numInports=2  catMethod=Horizontal
  A row 2 : simulink3/Signals & Systems/Matrix Concatenation  numInports=2  catMethod=Horizontal
  Ax : Product  Inputs=2  Multiplication=Matrix(*)  SaturateOnIntegerOverflow=on
  B : simulink3/Signals & Systems/Matrix Concatenation  numInports=2  catMethod=Vertical
  Bu : Product  Inputs=2  Multiplication=Matrix(*)  SaturateOnIntegerOverflow=on
  C : simulink3/Signals & Systems/Matrix Concatenation  numInports=2  catMethod=Horizontal
  Constant : Constant  Value=0
  Constant1 : Constant  Value=1
  Cx : Product  Inputs=2  Multiplication=Matrix(*)  SaturateOnIntegerOverflow=on
  Derivative : Derivative
  Gain : Gain  Gain=2  Multiplication=Element-wise(K.*u)  SaturateOnIntegerOverflow=on
  Gain1 : Gain  Gain=-28.84  Multiplication=Element-wise(K.*u)  SaturateOnIntegerOverflow=on
  Gain2 : Gain  Gain=1.776  Multiplication=Element-wise(K.*u)  SaturateOnIntegerOverflow=on
  Gain3 : Gain  Gain=-26.51  Multiplication=Element-wise(K.*u)  SaturateOnIntegerOverflow=on
  Gain4 : Gain  Gain=26.51  Multiplication=Element-wise(K.*u)  SaturateOnIntegerOverflow=on
  Integrator : Integrator  ExternalReset=none  InitialConditionSource=internal  InitialCondition=zeros(2,1)  LimitOutput=off  UpperSaturationLimit=inf  LowerSaturationLimit=-inf  ShowSaturationPort=off  ShowStatePort=off  AbsoluteTolerance=auto
  Math Function : Math  Operator=square  OutputSignalType=auto
  Math Function1 : Math  Operator=sqrt  OutputSignalType=auto
  Product : Product  Inputs=*/  Multiplication=Element-wise(.*)  SaturateOnIntegerOverflow=on
  Product1 : Product  Inputs=*/  Multiplication=Element-wise(.*)  SaturateOnIntegerOverflow=on
  Product2 : Product  Inputs=2  Multiplication=Element-wise(.*)  SaturateOnIntegerOverflow=on
  Sum : Sum  Inputs=|++  SaturateOnIntegerOverflow=on
  White Noise : RandomNumber  Mean=0  Variance=1  Seed=[44231]  SampleTime=tsamp
  VertVel : Outport  Port=1
  VertAcc : Outport  Port=2
  wires:
  Airspeed/1 -> Product1/2, Product/1
  RefLength/1 -> Product1/1, Product/2
  Product1/1 -> Gain/1
  Product/1 -> Math Function/1, Gain1/1, Gain2/1
  Gain/1 -> Math Function1/1
  Gain1/1 -> A row 1/1
  Gain2/1 -> C/1
  Math Function/1 -> Gain3/1, Gain4/1
  Gain3/1 -> A row 1/2
  Gain4/1 -> C/2
  Math Function1/1 -> Product2/1
  Product2/1 -> B/1
  Constant1/1 -> A row 2/1
  Constant/1 -> A row 2/2, B/2
  A row 1/1 -> A/1
  A row 2/1 -> A/2
  A/1 -> Ax/1
  B/1 -> Bu/1
  C/1 -> Cx/1
  Ax/1 -> Sum/1
  Sum/1 -> Integrator/1
  White Noise/1 -> Bu/2
  Bu/1 -> Sum/2
  Cx/1 -> VertVel/1, Derivative/1
  Derivative/1 -> VertAcc/1
  Intensity/1 -> Product2/2
  Integrator/1 -> Ax/2, Cx/2

== system tp333079/Atmosphere/Wind Shear/Zero Offset1 ==
  In : Inport  Port=1  PortDimensions=-1  SampleTime=-1  DataType=auto
      settings: SignalType=auto
  Abs : Abs  SaturateOnIntegerOverflow=on
  Constant : Constant  Value=tol
  Non-zero Sign : Subsystem  SimViewingDevice=off
      settings: Permissions=ReadWrite  RTWFcnNameOpts=Auto  RTWFileNameOpts=Auto
      mask Type: Non-zero sign
      mask Description: Sign function outputs 1 for input greater than or equal to 0, and -1 otherwise.
  Product : Product  Inputs=2  Multiplication=Element-wise(.*)  SaturateOnIntegerOverflow=on
  Switch : Switch  Threshold=tol
  Out : Outport  Port=1
  wires:
  In/1 -> Switch/1, Non-zero Sign/1(In), Abs/1
  Abs/1 -> Switch/2
  Non-zero Sign/1(Out) -> Product/1
  Constant/1 -> Product/2
  Product/1 -> Switch/3
  Switch/1 -> Out/1

== system tp333079/Atmosphere/Wind Shear/Zero Offset2 ==
  In : Inport  Port=1  PortDimensions=-1  SampleTime=-1  DataType=auto
      settings: SignalType=auto
  Abs : Abs  SaturateOnIntegerOverflow=on
  Constant : Constant  Value=tol
  Non-zero Sign : Subsystem  SimViewingDevice=off
      settings: Permissions=ReadWrite  RTWFcnNameOpts=Auto  RTWFileNameOpts=Auto
      mask Type: Non-zero sign
      mask Description: Sign function outputs 1 for input greater than or equal to 0, and -1 otherwise.
  Product : Product  Inputs=2  Multiplication=Element-wise(.*)  SaturateOnIntegerOverflow=on
  Switch : Switch  Threshold=tol
  Out : Outport  Port=1
  wires:
  Switch/1 -> Out/1
  Product/1 -> Switch/3
  Constant/1 -> Product/2
  Non-zero Sign/1(Out) -> Product/1
  Abs/1 -> Switch/2
  In/1 -> Abs/1, Non-zero Sign/1(In), Switch/1

== system tp333079/Complete Aircraft/6-DOF Aircraft Model (Body-frame EOM)/Aerodynamics ==
  note: Aerodynamic Loads
  note: Aerodynamic Coefficients
  note: Aerodynamic Parameters
  note: Outputs
  note: Inputs
  VelB : Inport  Port=1  PortDimensions=[3 1]  SampleTime=-1  DataType=auto
      settings: SignalType=auto
  WindB : Inport  Port=2  PortDimensions=[3 1]  SampleTime=-1  DataType=auto
      settings: SignalType=auto
  Rates : Inport  Port=3  PortDimensions=[3 1]  SampleTime=-1  DataType=auto
      settings: SignalType=auto
  WindRates : Inport  Port=4  PortDimensions=[3 1]  SampleTime=-1  DataType=auto
      settings: SignalType=auto
  AeroCon : Inport  Port=5  PortDimensions=[4 1]  SampleTime=-1  DataType=auto
      settings: SignalType=auto
  rho : Inport  Port=6  PortDimensions=1  SampleTime=-1  DataType=auto
      settings: SignalType=auto
  a : Inport  Port=7  PortDimensions=1  SampleTime=-1  DataType=auto
      settings: SignalType=auto
  Aerodynamic Force : aerosimlib/Aerodynamics/Aerodynamic Force  S=S
  Aerodynamic Moment : aerosimlib/Aerodynamics/Aerodynamic Moment  c=MAC  b=b  S=S
  Drag Coefficient : aerosimlib/Aerodynamics/Drag Coefficient  CL0=CLmind  CD0=CDmin  CDdf=CDdf  CDde=CDde  CDda=CDda  CDdr=CDdr  CDM=CDM  e=osw  b=b  S=S
  Dynamic Pressure : aerosimlib/Aerodynamics/Dynamic Pressure
  Lift Coefficient : aerosimlib/Aerodynamics/Lift Coefficient  CL0=CL0  CLalpha=CLa  CLdf=CLdf  CLde=CLde  CLalphadot=CLalphadot  CLq=CLq  CLM=CLM  c=MAC
  Mux : Mux  Inputs=6
  Pitch Moment Coefficient : aerosimlib/Aerodynamics/Pitch Moment Coefficient  Cm0=Cm0  Cma=Cma  Cmdf=Cmdf  Cmde=Cmde  Cmalphadot=Cmalphadot  Cmq=Cmq  CmM=CmM  c=MAC
  Roll Moment Coefficient : aerosimlib/Aerodynamics/Roll Moment Coefficient  Clbeta=Clbeta  Clda=Clda  Cldr=Cldr  Clp=Clp  Clr=Clr  b=b
  Side Force Coefficient : aerosimlib/Aerodynamics/Side Force Coefficient  CYbeta=CYbeta  CYda=CYda  CYdr=CYdr  CYp=CYp  CYr=CYr  b=b
  Sum : Sum  Inputs=|+-  SaturateOnIntegerOverflow=on
  Wind-axes Velocities : aerosimlib/Aerodynamics/Wind-axes Velocities  Vabnd=VaBnd  betabnd=BetaBnd  alphabnd=AlphaBnd
  Yaw Moment Coefficient : aerosimlib/Aerodynamics/Yaw Moment Coefficient  Cnbeta=Cnbeta  Cnda=Cnda  Cndr=Cndr  Cnp=Cnp  Cnr=Cnr  b=b
  Faero : Outport  Port=1
  Maero : Outport  Port=2
  AeroCoeff : Outport  Port=3
  VelW : Outport  Port=4
  Mach : Outport  Port=5
  pdyn : Outport  Port=6
  wires:
  VelB/1 -> Wind-axes Velocities/1
  WindB/1 -> Wind-axes Velocities/2
  a/1 -> Wind-axes Velocities/3
  Wind-axes Velocities/1 -> Lift Coefficient/1, Dynamic Pressure/1, Drag Coefficient/1, Side Force Coefficient/1, Pitch Moment Coefficient/1, Roll Moment Coefficient/1, Yaw Moment Coefficient/1, Aerodynamic Force/5, VelW/1
  rho/1 -> Dynamic Pressure/2
  AeroCon/1 -> Lift Coefficient/2, Drag Coefficient/2, Side Force Coefficient/2, Pitch Moment Coefficient/2, Roll Moment Coefficient/2, Yaw Moment Coefficient/2
  Wind-axes Velocities/2 -> Lift Coefficient/3, Pitch Moment Coefficient/3
  Wind-axes Velocities/3 -> Drag Coefficient/4, Pitch Moment Coefficient/5, Lift Coefficient/5, Mach/1
  Lift Coefficient/1 -> Aerodynamic Force/3, Drag Coefficient/3, Mux/3
  Drag Coefficient/1 -> Aerodynamic Force/1, Mux/1
  Side Force Coefficient/1 -> Aerodynamic Force/2, Mux/2
  Dynamic Pressure/1 -> Aerodynamic Force/4, Aerodynamic Moment/4, pdyn/1
  Roll Moment Coefficient/1 -> Aerodynamic Moment/1, Mux/4
  Pitch Moment Coefficient/1 -> Aerodynamic Moment/2, Mux/5
  Yaw Moment Coefficient/1 -> Aerodynamic Moment/3, Mux/6
  Aerodynamic Force/1 -> Faero/1
  Aerodynamic Moment/1 -> Maero/1
  Mux/1 -> AeroCoeff/1
  Rates/1 -> Sum/1
  WindRates/1 -> Sum/2
  Sum/1 -> Lift Coefficient/4, Side Force Coefficient/3, Pitch Moment Coefficient/4, Yaw Moment Coefficient/3, Roll Moment Coefficient/3
